simulink model "ind"  (R2023b)
settings: Solver=ode1  StartTime=0.0  StopTime=2  FixedStep=1e-6  RelTol=1e-3
undefined symbols (not defined in the file): B, j, Lm, Ls, Lsig, p, Rr, Rs, x
libraries: spsIdealSwitchLib x6, spsVoltageMeasurementLib x3, spsDCVoltageSourceLib x1, simulink x1, sps_lib x1
settings Model: Creator=user  LastModifiedBy=user

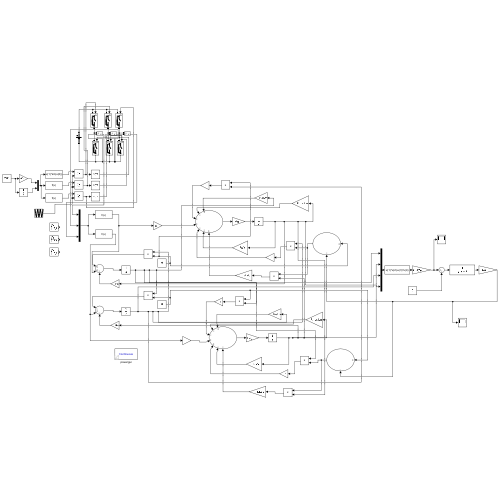
[thumbnail: Simulink's stored preview of the top-level diagram]
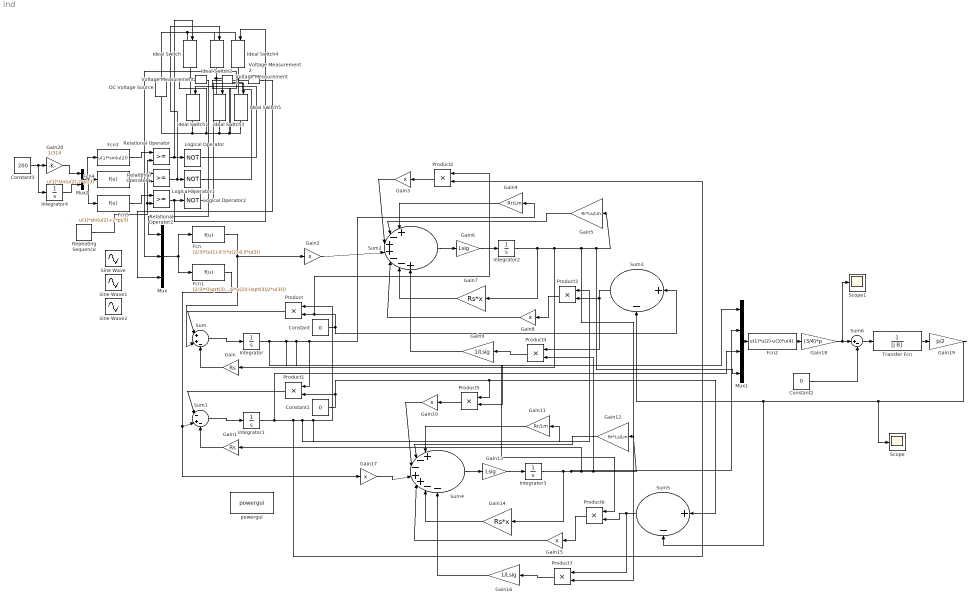
== system ind ==
  Constant : Constant  Value=0
  Constant1 : Constant  Value=0
  Constant2 : Constant  Value=0
  Constant3 : Constant  Value=200
  DC Voltage Source : spsDCVoltageSourceLib/DC Voltage Source  Amplitude=560  Measurements=None
  Fcn : Fcn  Expr=(2/3)*(u(1)-0.5*u(2)-0.5*u(3))
  Fcn1 : Fcn  Expr=(2/3)*((sqrt(3)/2*u(2))-(sqrt(3)/2*u(3)))
  Fcn2 : Fcn  Expr=u(1)*u(2)-u(3)*u(4)
  Fcn3 : Fcn  Expr=u(1)*sin(u(2))
  Fcn4 : Fcn  Expr=u(1)*sin(u(2)-2*pi/3)
  Fcn5 : Fcn  Expr=u(1)*sin(u(2)+2*pi/3)
  Gain : Gain  Gain=Rs
  Gain1 : Gain  Gain=Rs
  Gain{2..3,8,10,15,17} (6 alike) : Gain  Gain=x
  Gain11 : Gain  Gain=Rr/Lm
  Gain12 : Gain  Gain=Rr*Ls/Lm
  Gain13 : Gain  Gain=Lsig
  Gain14 : Gain  Gain=Rs*x
  Gain16 : Gain  Gain=1/Lsig
  Gain18 : Gain  Gain=(3/4)*p
  Gain19 : Gain  Gain=p/2
  Gain20 : Gain  Gain=1/314
  Gain4 : Gain  Gain=Rr/Lm
  Gain5 : Gain  Gain=Rr*Ls/Lm
  Gain6 : Gain  Gain=Lsig
  Gain7 : Gain  Gain=Rs*x
  Gain9 : Gain  Gain=1/Lsig
  Ideal Switch{,1..5} (6 alike) : spsIdealSwitchLib/Ideal Switch  Ron=0.001  Lon=0  IC=0  Rs=1e5  Cs=inf  Measurements=off
  Integrator{,1..4} (5 alike) : Integrator
  Logical Operator : Logic  Operator=NOT  AllPortsSameDT=off  OutDataTypeStr=boolean
  Logical Operator1 : Logic  Operator=NOT  AllPortsSameDT=off  OutDataTypeStr=boolean
  Logical Operator2 : Logic  Operator=NOT  AllPortsSameDT=off  OutDataTypeStr=boolean
  Mux : Mux  Inputs=3
  Mux1 : Mux
  Mux2 : Mux  Inputs=2
  Product{,1..7} (8 alike) : Product
  Relational Operator : RelationalOperator  OutDataTypeStr=boolean  RndMeth=Simplest  InputSameDT=off
  Relational Operator1 : RelationalOperator  OutDataTypeStr=boolean  RndMeth=Simplest  InputSameDT=off
  Relational Operator2 : RelationalOperator  OutDataTypeStr=boolean  RndMeth=Simplest  InputSameDT=off
  Repeating Sequence : simulink/Sources/Repeating Sequence  rep_seq_t=[0 0.25 0.5 0.75 1]*1/1050  rep_seq_y=[1 0 -1 0 1]
  Scope : Scope
  Scope1 : Scope
  Sine Wave : Sin  Amplitude=283  Frequency=2*pi*50  SampleTime=0
  Sine Wave1 : Sin  Amplitude=283  Frequency=2*pi*50  Phase=-(2/3)*pi  SampleTime=0
  Sine Wave2 : Sin  Amplitude=283  Frequency=2*pi*50  Phase=(2/3)*pi  SampleTime=0
  Sum : Sum  Inputs=|++-
  Sum1 : Sum  Inputs=|-+-
  Sum2 : Sum  Inputs=|+-++--+
  Sum3 : Sum  Inputs=|+-
  Sum4 : Sum  Inputs=|+--++--
  Sum5 : Sum  Inputs=|+-
  Sum6 : Sum  Inputs=|+-
  Transfer Fcn : TransferFcn  Denominator=[j B]  ParameterTunability=Unconstrained
  Voltage Measurement : spsVoltageMeasurementLib/Voltage Measurement  PhasorSimulation=off  OutputType=Complex  PSBequivalent=0
  Voltage Measurement1 : spsVoltageMeasurementLib/Voltage Measurement  PhasorSimulation=off  OutputType=Complex  PSBequivalent=0
  Voltage Measurement2 : spsVoltageMeasurementLib/Voltage Measurement  PhasorSimulation=off  OutputType=Complex  PSBequivalent=0
  powergui : sps_lib/powergui  Priority=1  SimulationMode=Continuous  SampleTime=50e-6  frequency=60  Iterations=50  frequencyindice=0  Pbase=100e6  ErrMax=1e-4  UnitsV=kV  UnitsW=MW  buscounter=0  FunctionMessages=off  echomessages=off  EnableUseOfTLC=off  CurrentSourceSwitches=off  DisableSnubberDevices=off  DisableRonSwitches=off  DisableVfSwitches=off  DisplayEquations=off  AutomaticDiscreteSolvers=off  SolverType=Tustin/Backward Euler (TBE)  Interpol=off  ExternalGateDelay=off  methode=off  Ts=100  x0status=blocks  SPID=on  SwTol=0  HookPort=off  NonlinearTolerance=1e-4  nMaxIteration=100  ContinueOnMaxIteration=off  RestoreLinks=warning  ResistiveCurrentMeasurement=off  Frange=[0:2:500]  Ylog=off  Xlog=on  ShowGrid=off  save=off  variable=ZData  structure=0  ZoomFFT=off  StartTime=0.0  cycles=1  DisplayStyle=1  fundamental=60  FreqAxis=off  MaxFrequency=1000  frequencyindicesteady=1  RmsSteady=1  display=off
  wires:
  Mux/1 -> Fcn1/1, Fcn/1
  Fcn/1 -> Gain2/1, Sum/2
  Constant/1 -> Product2/1, Product/2, Sum3/1
  Product/1 -> Sum/1
  Sum/1 -> Integrator/1
  Gain/1 -> Sum/3
  Gain1/1 -> Sum1/3
  Sum1/1 -> Integrator1/1
  Product1/1 -> Sum1/1
  Constant1/1 -> Product5/1, Sum5/1, Product1/2
  Fcn1/1 -> Gain17/1, Sum1/2
  Integrator1/1 -> Mux1/3, Product2/2, Product3/1, Gain11/1, Product/1
  Integrator/1 -> Mux1/1, Product6/1, Product5/2, Gain4/1, Product1/1
  Gain2/1 -> Sum2/4
  Sum2/1 -> Gain6/1
  Gain6/1 -> Integrator2/1
  Product2/1 -> Gain3/1
  Gain3/1 -> Sum2/3
  Gain5/1 -> Sum2/2
  Gain4/1 -> Sum2/1
  Gain7/1 -> Sum2/6
  Gain9/1 -> Sum2/7
  Gain8/1 -> Sum2/5
  Integrator2/1 -> Gain/1, Product7/2, Mux1/4, Gain5/1, Gain7/1
  Product3/1 -> Gain8/1
  Product4/1 -> Gain9/1
  Sum3/1 -> Product4/1, Product3/2
  Sum5/1 -> Product6/2, Product7/1
  Product7/1 -> Gain16/1
  Product6/1 -> Gain15/1
  Gain15/1 -> Sum4/5
  Gain16/1 -> Sum4/7
  Gain14/1 -> Sum4/6
  Gain11/1 -> Sum4/1
  Gain12/1 -> Sum4/2
  Gain10/1 -> Sum4/3
  Product5/1 -> Gain10/1
  Gain13/1 -> Integrator3/1
  Sum4/1 -> Gain13/1
  Gain17/1 -> Sum4/4
  Integrator3/1 -> Gain14/1, Mux1/2, Gain1/1, Gain12/1, Product4/2
  Mux1/1 -> Fcn2/1
  Fcn2/1 -> Gain18/1
  Sum6/1 -> Transfer Fcn/1
  Transfer Fcn/1 -> Gain19/1
  Constant2/1 -> Sum6/2
  Gain18/1 -> Scope1/1, Sum6/1
  Gain19/1 -> Scope/1, Sum3/2, Sum5/2
  Constant3/1 -> Integrator4/1, Gain20/1
  Gain20/1 -> Mux2/1
  Integrator4/1 -> Mux2/2
  Mux2/1 -> Fcn5/1, Fcn4/1, Fcn3/1
  Fcn3/1 -> Relational Operator/1
  Fcn5/1 -> Relational Operator2/1
  Fcn4/1 -> Relational Operator1/1
  Repeating Sequence/1 -> Relational Operator/2, Relational Operator1/2, Relational Operator2/2
  Voltage Measurement/1 -> Mux/1
  Voltage Measurement1/1 -> Mux/2
  Voltage Measurement2/1 -> Mux/3
  Relational Operator/1 -> Ideal Switch/1, Logical Operator/1
  Relational Operator1/1 -> Ideal Switch2/1, Logical Operator1/1
  Relational Operator2/1 -> Ideal Switch4/1, Logical Operator2/1
  Logical Operator/1 -> Ideal Switch1/1
  Logical Operator1/1 -> Ideal Switch3/1
  Logical Operator2/1 -> Ideal Switch5/1
  connections:
  Ideal Switch3/LConn1 -- Voltage Measurement1/LConn1 -- Ideal Switch2/RConn1
  Ideal Switch5/LConn1 -- Voltage Measurement2/LConn1 -- Ideal Switch4/RConn1
  Ideal Switch1/LConn1 -- Voltage Measurement/LConn1 -- Ideal Switch/RConn1
  DC Voltage Source/RConn1 -- Ideal Switch4/LConn1 -- Ideal Switch2/LConn1 -- Ideal Switch/LConn1
  Ideal Switch1/RConn1 -- Voltage Measurement/LConn2 -- Ideal Switch5/RConn1 -- Voltage Measurement2/LConn2 -- Voltage Measurement1/LConn2 -- Ideal Switch3/RConn1 -- DC Voltage Source/LConn1
